simulink model "actuator"  (R2025b)
settings: Solver=FixedStepDiscrete  StartTime=0.0  StopTime=10.0  RelTol=1e-3  EnableMultiTasking=on
settings Model: Creator=karadeli  LastModifiedBy=karadeli
settings SolverCC: AutoInsertRateTranBlk=on
settings OptimizationCC: DefaultParameterBehavior=Inlined  UseDivisionForNetSlopeComputation=on  GainParamInheritBuiltInType=on  UseFloatMulNetSlope=on  InlineInvariantSignals=on  PassReuseOutputArgsAs=Individual arguments  ZeroExternalMemoryAtStartup=off  ZeroInternalMemoryAtStartup=off  NoFixptDivByZeroProtection=on  EfficientFloat2IntCast=on  LifeSpan=1  OptimizeBlockOrder=speed  DifferentSizesBufferReuse=on  EfficientTunableParamExpr=on
settings DebuggingCC: ParameterTunabilityLossMsg=error
settings HardwareCC: ProdBitPerPointer=32.0  ProdBitPerSizeT=32.0  ProdBitPerPtrDiffT=32.0  ProdLargestAtomicInteger=Long  ProdLargestAtomicFloat=Double  ProdWordSize=32.0  ProdLongLongMode=on  ProdHWDeviceType=ARM Compatible->ARM Cortex-M
settings SFSimCC: MATLABDynamicMemAlloc=off
settings RTWCC: SystemTargetFile=ert.tlc  GenCodeOnly=on  TemplateMakefile=ert_default_tmf  TargetLang=C++  Description=Embedded Coder
settings CodeAppCC: ForceParamTrailComments=on  IgnoreCustomStorageClasses=off  OperatorAnnotations=on  SimulinkDataObjDesc=on  SFDataObjDesc=on  InsertBlockDesc=on
settings ERTTargetCC: RootIOFormat=Structure reference  ERTCustomFileTemplate=example_file_process.tlc  ERTFilePackagingFormat=CompactWithDataFile  TargetLangStandard=C++11 (ISO)  GenerateSampleERTMain=on  IncludeMdlTerminateFcn=off  CombineSignalStateStructs=on  SuppressErrorStatus=on  SupportAbsoluteTime=off  CodeInterfacePackaging=C++ class  SubcomponentCodeInterfacePackaging=C++ class  SupportComplex=off

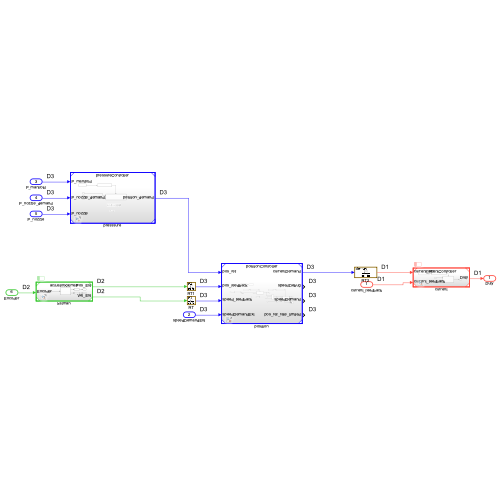
[thumbnail: Simulink's stored preview of the top-level diagram]
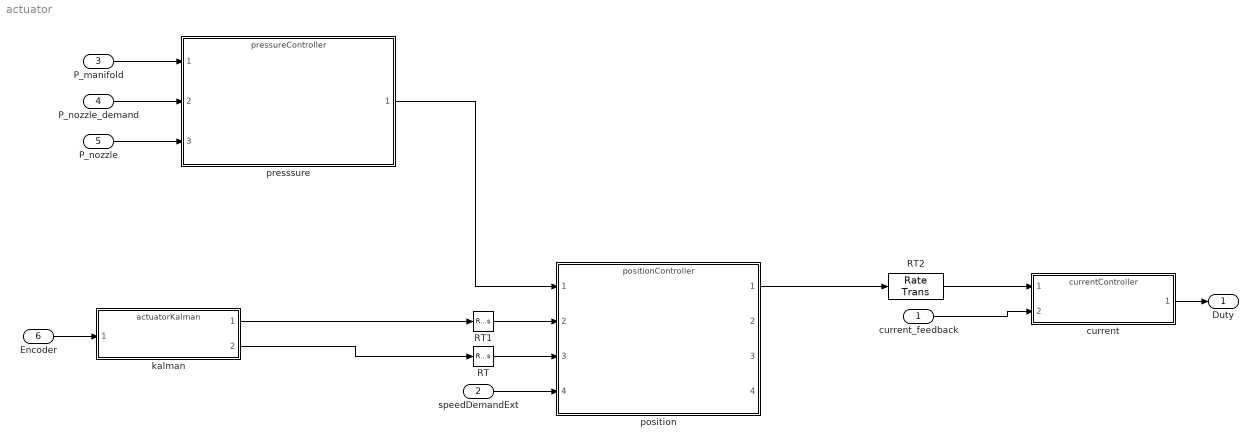
== system actuator ==
  current_feedback : Inport
  speedDemandExt : Inport  Port=2
  P_manifold : Inport  Port=3
  P_nozzle_demand : Inport  Port=4
  P_nozzle : Inport  Port=5
  Encoder : Inport  Port=6
  RT : RateTransition  Deterministic=off  OutPortSampleTime=0.001
  RT1 : RateTransition  Deterministic=off  OutPortSampleTime=0.001
  RT2 : RateTransition  Deterministic=off  OutPortSampleTime=0.001/8
  current : ModelReference  ModelNameDialog=currentController.slx  SimulationMode=Normal  ScheduleRates=on  ScheduleRatesWith=Schedule Editor  ModelReferenceVersion=1.110
  kalman : ModelReference  ModelNameDialog=actuatorKalman.slx  SimulationMode=Normal  ScheduleRates=on  ScheduleRatesWith=Schedule Editor  ModelReferenceVersion=1.27
  position : ModelReference  ModelNameDialog=positionController.slx  SimulationMode=Normal  ModelReferenceVersion=1.44
  presssure : ModelReference  ModelNameDialog=pressureController.slx  SimulationMode=Normal  ModelReferenceVersion=1.32
  Duty : Outport
  wires:
  current_feedback/1 -> current/2
  current/1 -> Duty/1
  speedDemandExt/1 -> position/4
  P_manifold/1 -> presssure/1
  P_nozzle_demand/1 -> presssure/2
  P_nozzle/1 -> presssure/3
  presssure/1 -> position/1
  position/1 -> RT2/1
  Encoder/1 -> kalman/1
  RT2/1 -> current/1
  kalman/2 -> RT/1
  kalman/1 -> RT1/1
  RT/1 -> position/3
  RT1/1 -> position/2
